simulink model "picam_lanedepart"  (R2017a)
settings: Solver=FixedStepAuto  StartTime=0.0  StopTime=10.0  RelTol=1e-3  EnableMultiTasking=on
undefined symbols (not defined in the file or in its folder): gray, strel
libraries: visiontextngfix x4, visionsinks x1, visionmorphops x1, dspvision x1, visiongeotforms x1, embdlinuxlib x1
settings Model: Creator=Vincent  LastModifiedBy=Vincent
settings SolverCC: PositivePriorityOrder=on
settings OptimizationCC: PassReuseOutputArgsThreshold=0  MaxStackSize=64
settings DebuggingCC: ParameterTunabilityLossMsg=error
settings HardwareCC: ProdBitPerPointer=32  ProdBitPerSizeT=32  ProdBitPerPtrDiffT=32  ProdLargestAtomicInteger=Long  ProdLargestAtomicFloat=Double  ProdWordSize=32  ProdHWDeviceType=ARM Compatible->ARM Cortex  UseEmbeddedCoderFeatures=off
settings SFSimCC: MATLABDynamicMemAlloc=off
settings RTWCC: SystemTargetFile=ert.tlc  HardwareBoard=Raspberry Pi  TLCOptions="-aInlineSetEventsForThisBaseRateFcn=TLC_FALSE -aSuppressMultiTaskScheduler=TLC_FALSE  -aRateBasedStepFcn=0"  TemplateMakefile=ert_default_tmf  Description=Embedded Coder  GenerateReport=on  Toolchain=GNU GCC Raspberry Pi  LaunchReport=on
settings CodeAppCC: ForceParamTrailComments=on  OperatorAnnotations=on  MATLABSourceComments=on
settings ERTTargetCC: ERTCustomFileBanners=off  SupportContinuousTime=on  SupportNonInlinedSFcns=on  RemoveResetFunc=off  SupportVariableSizeSignals=on  ModelStepFunctionPrototypeControlCompliant=off

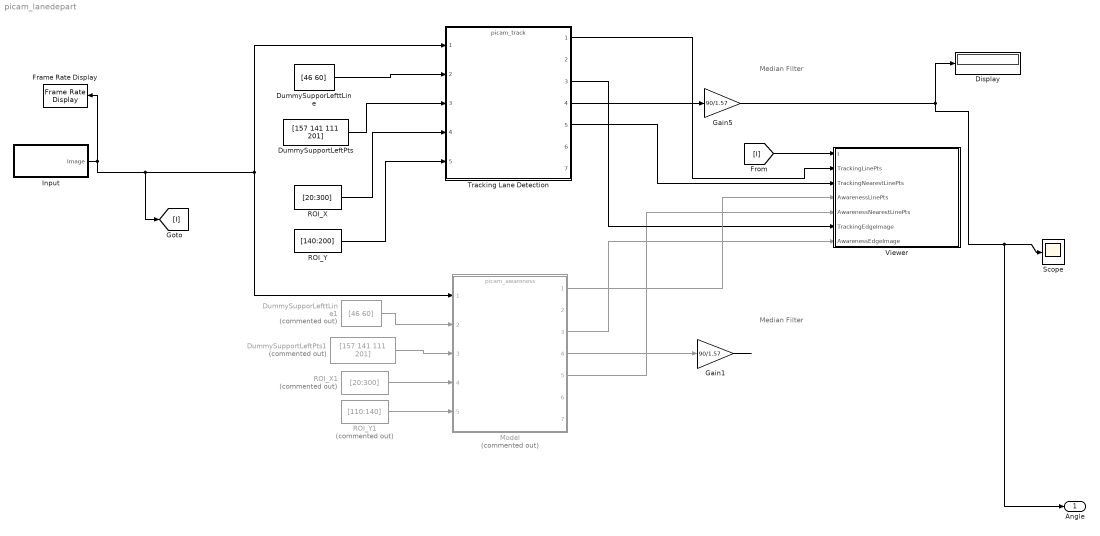
== system picam_lanedepart ==
  note: Median Filter
  note: Median Filter
  Display : Display
  DummySupporLefttLine : Constant  Value=[46 60]  VectorParams1D=off  OutDataTypeStr=double
  DummySupporLefttLine1 : Constant  Commented=on  Value=[46 60]  VectorParams1D=off  OutDataTypeStr=double
  DummySupportLeftPts : Constant  Value=[157 141 111 201]  OutDataTypeStr=double
  DummySupportLeftPts1 : Constant  Commented=on  Value=[157 141 111 201]  OutDataTypeStr=double
  Frame Rate Display : visionsinks/Frame Rate Display  UpdateRate=10
      settings: SourceProductName=Computer Vision System Toolbox  SourceProductBaseCode=VP
  Gain1 : Gain  Gain=90/1.57
  Gain5 : Gain  Gain=90/1.57
  "Input " : Subsystem
  Model : ModelReference  Commented=on  ModelNameDialog=picam_awareness.slx  SimulationMode=Normal  ModelReferenceVersion=1.333
  ROI_X : Constant  Value=[20:300]  LockScale=on
  ROI_X1 : Constant  Commented=on  Value=[20:300]  LockScale=on
  ROI_Y : Constant  Value=[140:200]  LockScale=on
  ROI_Y1 : Constant  Commented=on  Value=[110:140]  LockScale=on
  Scope : Scope
  Tracking Lane Detection : ModelReference  ModelNameDialog=picam_track.slx  SimulationMode=Normal  ModelReferenceVersion=1.6
  Viewer : Subsystem
  Angle : Outport
  wires:
  ROI_X1/1 -> Model/4
  Model/5 -> Viewer/5(AwarenessNearestLinePts)
  DummySupporLefttLine/1 -> Tracking Lane Detection/2
  Model/3 -> Viewer/7(AwarenessEdgeImage)
  DummySupporLefttLine1/1 -> Model/2
  ROI_X/1 -> Tracking Lane Detection/4
  ? -> ?
  Tracking Lane Detection/3 -> Viewer/6(TrackingEdgeImage)
  Tracking Lane Detection/1 -> Viewer/2(TrackingLinePts)
  Model/1 -> Viewer/4(AwarenessLinePts)
  DummySupportLeftPts1/1 -> Model/3
  "Input "/1(Image) -> [I], Tracking Lane Detection/1, Model/1, Frame Rate Display/1
  ROI_Y/1 -> Tracking Lane Detection/5
  Tracking Lane Detection/5 -> Viewer/3(TrackingNearestLinePts)
  [I] -> Viewer/1(I)
  Model/4 -> Gain1/1
  DummySupportLeftPts/1 -> Tracking Lane Detection/3
  ROI_Y1/1 -> Model/5
  Gain5/1 -> Display/1, Angle/1, Scope/1
  Tracking Lane Detection/4 -> Gain5/1
  Gain1/1 -> ?

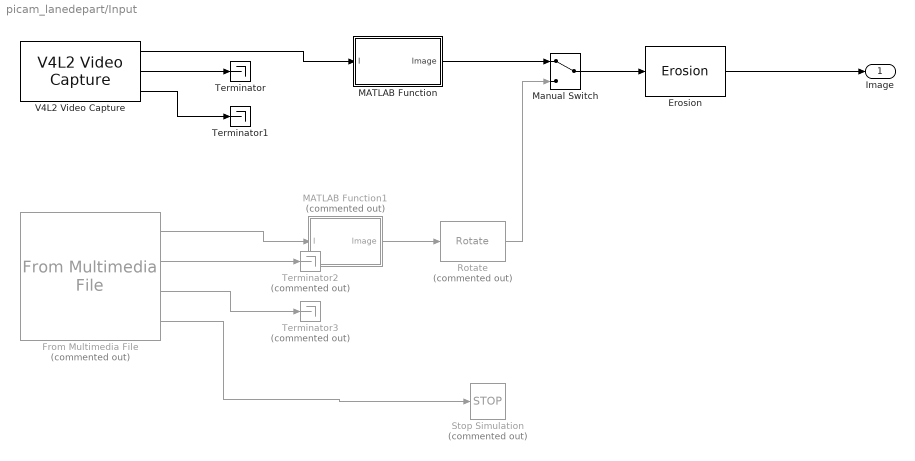
== system picam_lanedepart/Input  ==
  Erosion : visionmorphops/Erosion  nhoodsrc=Specify via dialog  strel=strel('square',4)
      settings: SourceProductName=Computer Vision System Toolbox  SourceProductBaseCode=VP
  From Multimedia File : dspvision/From Multimedia File  Commented=on  inputFilename=/Users/Vincent/Documents/GitHub/AMBD/testing_src/1.StrangeWay.mov  loop=on  numPlays=inf  outputStreams=Video only  videoDataType=uint8  audioDataType=int16  inheritSampleTime=off  userDefinedSampleTime=0.025  noAudioOutput=off  isIntensityVideo=off  fourcc=YCbCr 4:2:2  colorVideoFormat=One multidimensional signal  outputEOF=on  dataOrg=Column-major  audioFrameSize=1024  computeAudioFrameSize=off  outSamplingMode=Sample based
      settings: SourceProductBaseCode=VP
  MATLAB Function : MATLAB Function  TreatAsAtomicUnit=on
  MATLAB Function1 : MATLAB Function  Commented=on  TreatAsAtomicUnit=on
  Manual Switch : ManualSwitch
  Rotate : visiongeotforms/Rotate  Commented=on  outSizeR=Expanded to fit rotated input image  src_angle=Specify via dialog  unit_angle=Degrees  angle=pi  maxAngle=pi  dispImage=Top-left corner  method=Table lookup  fillVal=0  interpMethod=Bilinear  prodOutputMode=Binary point scaling  prodOutputWordLength=32  prodOutputFracLength=10  roundingMode=Nearest  overflowMode=on
      settings: SourceProductName=Computer Vision System Toolbox
  Stop Simulation : Stop  Commented=on
  Terminator : Terminator
  Terminator1 : Terminator
  Terminator2 : Terminator  Commented=on
  Terminator3 : Terminator  Commented=on
  V4L2 Video Capture : embdlinuxlib/V4L2 Video Capture  m_devName='/dev/video0'  roi=[0, 0, 640, 480]  imSizeSelection=320x240  imSize=[640, 480]  pixelFormat=YCbCr 4:2:2  pixelOrder=Planar  sampleTime=1/40  simOutput=Colorbars  blockPlatform=Raspberry Pi
  Image : Outport
  wires:
  V4L2 Video Capture/2 -> Terminator/1
  V4L2 Video Capture/3 -> Terminator1/1
  V4L2 Video Capture/1 -> MATLAB Function/1(I)
  From Multimedia File/2 -> Terminator2/1
  From Multimedia File/3 -> Terminator3/1
  From Multimedia File/1 -> MATLAB Function1/1(I)
  From Multimedia File/4 -> Stop Simulation/1
  MATLAB Function1/1(Image) -> Rotate/1
  MATLAB Function/1(Image) -> Manual Switch/1
  Manual Switch/1 -> Erosion/1
  Erosion/1 -> Image/1
  Rotate/1 -> Manual Switch/2

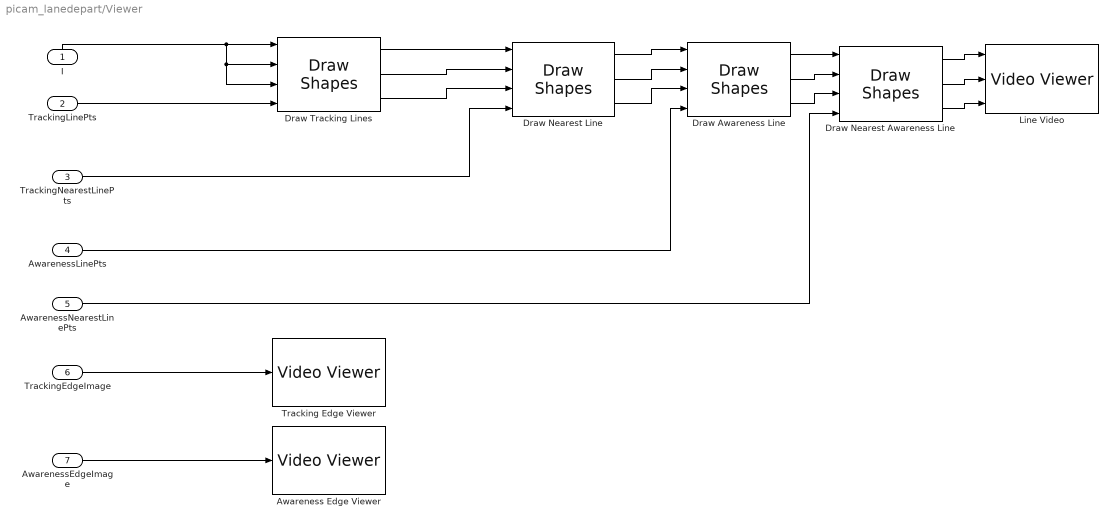
== system picam_lanedepart/Viewer ==
  I : Inport  OutDataTypeStr=uint8
  TrackingLinePts : Inport  Port=2
  TrackingNearestLinePts : Inport  Port=3
  AwarenessLinePts : Inport  Port=4
  AwarenessNearestLinePts : Inport  Port=5
  TrackingEdgeImage : Inport  Port=6
  AwarenessEdgeImage : Inport  Port=7
  Awareness Edge Viewer : VideoViewer  FigPos=[863 724 418 304]
  Draw Awareness Line : visiontextngfix/Draw Shapes  shape=Lines  fill=off  lineWidth=2  fillClrSource=Specify via dialog  display=User-specified value  intensity=200  color=[200 255 100]  opacity=0.6  viewport=Entire image  antialiasing=on  inType=Obsolete  imagePorts=Separate color signals  prodOutputMode=Binary point scaling  prodOutputWordLength=32  prodOutputFracLength=14  memoryMode=Specify word length  memoryWordLength=16  memoryFracLength=14  roundingMode=Floor  overflowMode=off
      settings: SourceProductName=Computer Vision System Toolbox  LockScale=on
  Draw Nearest Awareness Line : visiontextngfix/Draw Shapes  shape=Lines  fill=off  lineWidth=2  fillClrSource=Specify via dialog  display=User-specified value  intensity=200  color=[200 0 0]  opacity=0.6  viewport=Entire image  antialiasing=on  inType=Obsolete  imagePorts=Separate color signals  prodOutputMode=Binary point scaling  prodOutputWordLength=32  prodOutputFracLength=14  memoryMode=Specify word length  memoryWordLength=16  memoryFracLength=14  roundingMode=Floor  overflowMode=off
      settings: SourceProductName=Computer Vision System Toolbox  LockScale=on
  Draw Nearest Line : visiontextngfix/Draw Shapes  shape=Lines  fill=off  lineWidth=2  fillClrSource=Specify via dialog  display=User-specified value  intensity=200  color=[200 0 0]  opacity=0.6  viewport=Entire image  antialiasing=on  inType=Obsolete  imagePorts=Separate color signals  prodOutputMode=Binary point scaling  prodOutputWordLength=32  prodOutputFracLength=14  memoryMode=Specify word length  memoryWordLength=16  memoryFracLength=14  roundingMode=Floor  overflowMode=off
      settings: SourceProductName=Computer Vision System Toolbox  LockScale=on
  Draw Tracking Lines : visiontextngfix/Draw Shapes  shape=Lines  fill=off  lineWidth=1  fillClrSource=Specify via dialog  display=User-specified value  intensity=200  color=[200 255 100]  opacity=0.6  viewport=Entire image  antialiasing=on  inType=Obsolete  imagePorts=Separate color signals  prodOutputMode=Binary point scaling  prodOutputWordLength=32  prodOutputFracLength=14  memoryMode=Specify word length  memoryWordLength=16  memoryFracLength=14  roundingMode=Floor  overflowMode=off
      settings: SourceProductName=Computer Vision System Toolbox  LockScale=on
  Line Video : VideoViewer  imagePorts=separate color signals  colormapValue=gray(256)  FigPos=[61 592.4 417.6 304]
  Tracking Edge Viewer : VideoViewer  FigPos=[575 751 418 304]
  wires:
  I/1 -> Draw Tracking Lines/3, Draw Tracking Lines/2, Draw Tracking Lines/1
  Draw Tracking Lines/1 -> Draw Nearest Line/1
  Draw Tracking Lines/2 -> Draw Nearest Line/2
  Draw Tracking Lines/3 -> Draw Nearest Line/3
  Draw Nearest Line/1 -> Draw Awareness Line/1
  Draw Nearest Line/2 -> Draw Awareness Line/2
  Draw Nearest Line/3 -> Draw Awareness Line/3
  Draw Awareness Line/1 -> Draw Nearest Awareness Line/1
  Draw Awareness Line/2 -> Draw Nearest Awareness Line/2
  Draw Awareness Line/3 -> Draw Nearest Awareness Line/3
  Draw Nearest Awareness Line/1 -> Line Video/1
  Draw Nearest Awareness Line/2 -> Line Video/2
  Draw Nearest Awareness Line/3 -> Line Video/3
  TrackingLinePts/1 -> Draw Tracking Lines/4
  TrackingNearestLinePts/1 -> Draw Nearest Line/4
  AwarenessLinePts/1 -> Draw Awareness Line/4
  AwarenessNearestLinePts/1 -> Draw Nearest Awareness Line/4
  TrackingEdgeImage/1 -> Tracking Edge Viewer/1
  AwarenessEdgeImage/1 -> Awareness Edge Viewer/1

== matlab function picam_lanedepart/Input /MATLAB Function1 ==
  data: I input; Image output
function Image = Flip(I)

Image = imrotate(I,180,'bilinear');

== matlab function picam_lanedepart/Input /MATLAB Function ==
  data: I input; Image output
function Image = FlipAndRotate(I)
Image = imrotate(I,90,'bilinear');
Image = flip(Image,2);
